simulink model "Vehicle_model_without_controller"  (R2024b)
settings: Solver=FixedStepAuto  StartTime=0  StopTime=1370  FixedStep=1  RelTol=1e-3
values from neighbouring files (symbols this model uses):
  Eff_2DLUT = [0.5417 0.5417 0.7 0.7908 0.8336 0.8638 0.9083 0.9278 0.9349 0.9437 0.9503 0.9475 ... (360 elements, 18x20)]    [MC_PM49.mat]    (also in motor_map_data.mat = [0.851419264642 0.851644655878 0.85189721745 0.852178660652 )
  Max_torque_1DLUT = [274.4 274.4 274.4 274.4 233.8 187 155.9 133.6 116.9 103.9 93.5 85 ... (18 elements, 18x1)]    [MC_PM49.mat]    (also in motor_map_data.mat = [300 300 300 300 300 300 300 300 300 300 300 290.819486922 .)
  motor_rpm = [0 500 1000 1500 2000 2500 3000 3500 4000 4500 5000 5500 ... (18 elements, 1x18)]    [MC_PM49.mat]    (also in motor_map_data.mat = [0 200 400 600 800 1000 1200 1400 1600 1800 2000 2200 ... (6)
  motor_trq = [-176.4 -156.8 -137.2 -117.6 -98 -78.4 -58.8 -39.2 -19.6 0 19.6 39.2 ... (20 elements, 20x1)]    [MC_PM49.mat]    (also in motor_map_data.mat = [-300 -288 -276 -264 -252 -240 -228 -216 -204 -192 -180 -168)
undefined symbols (not defined in the file or in its folder): DiscIntNeverNeededParam, eng_fuel_gps, eng_rpm_bp, eng_Tmax_tab, eng_tq_bp, LHV_kJ_g
settings Model: Creator=hesha  LastModifiedBy=yashp

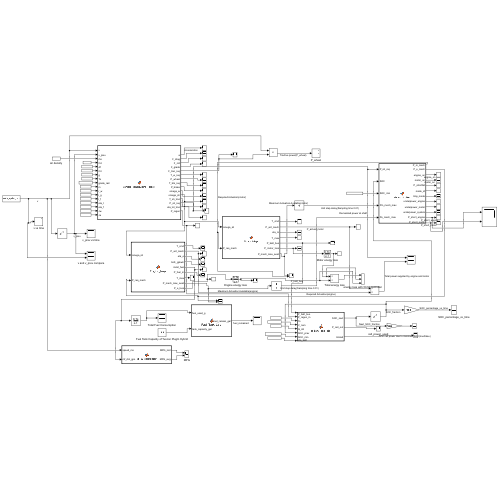
[thumbnail: Simulink's stored preview of the top-level diagram]
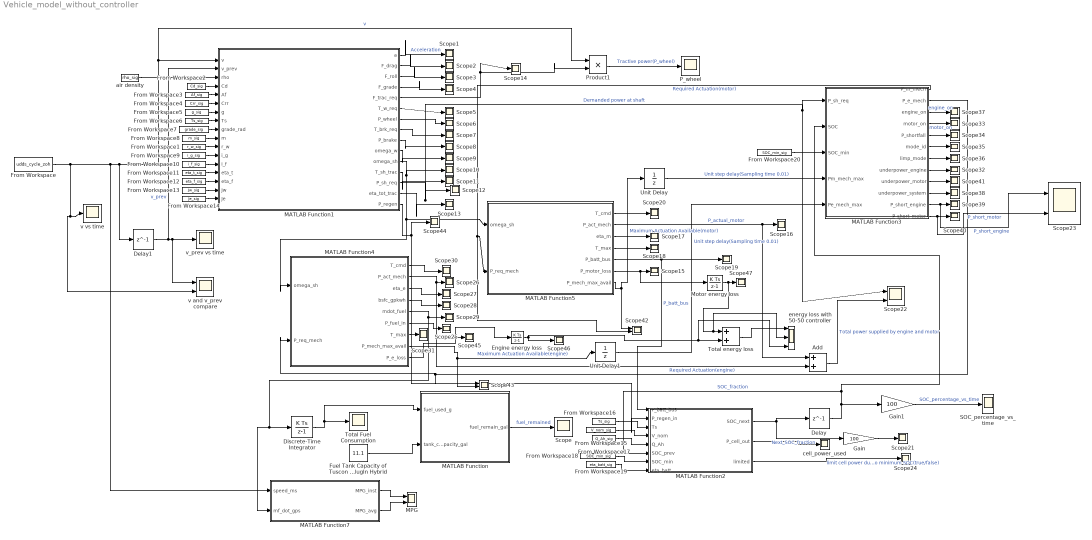
== system Vehicle_model_without_controller ==
  Add : Sum
  Delay : Delay  DelayLength=1  InitialCondition=0.8  InputProcessing=Columns as channels (frame based)
  Delay1 : Delay  DelayLength=1  InputProcessing=Columns as channels (frame based)
  Discrete-Time Integrator : DiscreteIntegrator  SampleTime=-1  ICPrevOutput=DiscIntNeverNeededParam  ICPrevScaledInput=DiscIntNeverNeededParam
  Engine energy loss : DiscreteIntegrator  SampleTime=-1  ICPrevOutput=DiscIntNeverNeededParam  ICPrevScaledInput=DiscIntNeverNeededParam
  From Workspace : FromWorkspace  VariableName=udds_cycle_zoh  OutDataTypeStr=double  SampleTime=-1  Interpolate=off  OutputAfterFinalValue=Setting to zero
  From Workspace1 : FromWorkspace  VariableName=r_w_sig  OutDataTypeStr=double  SampleTime=1  Interpolate=off  OutputAfterFinalValue=Setting to zero
  From Workspace10 : FromWorkspace  VariableName=i_f_sig  OutDataTypeStr=double  SampleTime=1  Interpolate=off  OutputAfterFinalValue=Setting to zero
  From Workspace11 : FromWorkspace  VariableName=eta_t_sig  OutDataTypeStr=double  SampleTime=1  Interpolate=off  OutputAfterFinalValue=Setting to zero
  From Workspace12 : FromWorkspace  VariableName=eta_f_sig  OutDataTypeStr=double  SampleTime=1  Interpolate=off  OutputAfterFinalValue=Setting to zero
  From Workspace13 : FromWorkspace  VariableName=Jw_sig  OutDataTypeStr=double  SampleTime=1  Interpolate=off  OutputAfterFinalValue=Setting to zero
  From Workspace14 : FromWorkspace  VariableName=Je_sig  OutDataTypeStr=double  SampleTime=1  Interpolate=off  OutputAfterFinalValue=Setting to zero
  From Workspace15 : FromWorkspace  VariableName=V_nom_sig  OutDataTypeStr=double  SampleTime=1  Interpolate=off  OutputAfterFinalValue=Setting to zero
  From Workspace16 : FromWorkspace  VariableName=Ts_sig  OutDataTypeStr=double  SampleTime=1  Interpolate=off  OutputAfterFinalValue=Setting to zero
  From Workspace17 : FromWorkspace  VariableName=Q_Ah_sig  OutDataTypeStr=double  SampleTime=1  Interpolate=off  OutputAfterFinalValue=Setting to zero
  From Workspace18 : FromWorkspace  VariableName=SOC_min_sig  OutDataTypeStr=double  SampleTime=1  Interpolate=off  OutputAfterFinalValue=Setting to zero
  From Workspace19 : FromWorkspace  VariableName=eta_batt_sig  OutDataTypeStr=double  SampleTime=1  Interpolate=off  OutputAfterFinalValue=Setting to zero
  From Workspace2 : FromWorkspace  VariableName=Cd_sig  OutDataTypeStr=double  SampleTime=1  Interpolate=off  OutputAfterFinalValue=Setting to zero
  From Workspace20 : FromWorkspace  VariableName=SOC_min_sig  OutDataTypeStr=double  SampleTime=1  Interpolate=off  OutputAfterFinalValue=Setting to zero
  From Workspace3 : FromWorkspace  VariableName=Af_sig  OutDataTypeStr=double  SampleTime=1  Interpolate=off  OutputAfterFinalValue=Setting to zero
  From Workspace4 : FromWorkspace  VariableName=Crr_sig  OutDataTypeStr=double  SampleTime=1  Interpolate=off  OutputAfterFinalValue=Setting to zero
  From Workspace5 : FromWorkspace  VariableName=g_sig  OutDataTypeStr=double  SampleTime=1  Interpolate=off  OutputAfterFinalValue=Setting to zero
  From Workspace6 : FromWorkspace  VariableName=Ts_sig  OutDataTypeStr=double  SampleTime=1  Interpolate=off  OutputAfterFinalValue=Setting to zero
  From Workspace7 : FromWorkspace  VariableName=grade_sig  OutDataTypeStr=double  SampleTime=1  Interpolate=off  OutputAfterFinalValue=Setting to zero
  From Workspace8 : FromWorkspace  VariableName=m_sig  OutDataTypeStr=double  SampleTime=1  Interpolate=off  OutputAfterFinalValue=Setting to zero
  From Workspace9 : FromWorkspace  VariableName=i_g_sig  OutDataTypeStr=double  SampleTime=1  Interpolate=off  OutputAfterFinalValue=Setting to zero
  Fuel Tank Capacity of Tuscon PlugIn Hybrid : Constant  Value=11.1
  Gain : Gain  Gain=100
  Gain1 : Gain  Gain=100
  MATLAB Function : MATLAB Function  TreatAsAtomicUnit=on
  MATLAB Function1 : MATLAB Function  TreatAsAtomicUnit=on
  MATLAB Function2 : MATLAB Function  TreatAsAtomicUnit=on
  MATLAB Function3 : MATLAB Function  TreatAsAtomicUnit=on
  MATLAB Function4 : MATLAB Function  TreatAsAtomicUnit=on
  MATLAB Function5 : MATLAB Function  TreatAsAtomicUnit=on
  MATLAB Function7 : MATLAB Function  TreatAsAtomicUnit=on
  MPG : Scope  NumInputPorts=2
  Motor energy loss : DiscreteIntegrator  SampleTime=-1  ICPrevOutput=DiscIntNeverNeededParam  ICPrevScaledInput=DiscIntNeverNeededParam
  P_wheel : Scope
  Product1 : Product
  SOC_percentage_vs_time : Scope
  Scope{,1..21,24..41,44..47} (44 alike) : Scope
  Scope{22..23,42..43} (4 alike) : Scope  NumInputPorts=2
  Total Fuel Consumption : Scope
  Total energy loss : Sum
  Unit Delay : UnitDelay  SampleTime=-1  HasFrameUpgradeWarning=on
  Unit Delay1 : UnitDelay  SampleTime=-1  HasFrameUpgradeWarning=on
  air density : FromWorkspace  VariableName=rho_sig  OutDataTypeStr=double  SampleTime=1  Interpolate=off  OutputAfterFinalValue=Setting to zero
  cell_power_used : Scope
  energy loss with 50-50 controller : Scope  NumInputPorts=3
  v and v_prev compare : Scope  NumInputPorts=2
  v vs time : Scope
  v_prev vs time : Scope
  wires:
  From Workspace/1 -> v and v_prev compare/2, v vs time/1, MATLAB Function7/1(speed_ms), Product1/1, MATLAB Function1/1(v), Delay1/1  "v"
  air density/1 -> MATLAB Function1/3(rho)
  From Workspace2/1 -> MATLAB Function1/4(Cd)
  From Workspace3/1 -> MATLAB Function1/5(Af)
  From Workspace4/1 -> MATLAB Function1/6(Crr)
  From Workspace5/1 -> MATLAB Function1/7(g)
  From Workspace6/1 -> MATLAB Function1/8(Ts)
  From Workspace8/1 -> MATLAB Function1/10(m)
  Delay1/1 -> MATLAB Function1/2(v_prev), v_prev vs time/1, v and v_prev compare/1  "v_prev"
  MATLAB Function1/5(F_trac_req) -> Scope14/1, Product1/2
  Product1/1 -> P_wheel/1  "Tractive power(P_wheel)"
  MATLAB Function1/1(a) -> Scope1/1  "Acceleration"
  From Workspace1/1 -> MATLAB Function1/11(r_w)
  From Workspace9/1 -> MATLAB Function1/12(i_g)
  From Workspace10/1 -> MATLAB Function1/13(i_f)
  From Workspace11/1 -> MATLAB Function1/14(eta_t)
  From Workspace12/1 -> MATLAB Function1/15(eta_f)
  From Workspace13/1 -> MATLAB Function1/16(Jw)
  From Workspace14/1 -> MATLAB Function1/17(Je)
  MATLAB Function1/2(F_drag) -> Scope2/1
  MATLAB Function1/3(F_roll) -> Scope3/1
  MATLAB Function1/4(F_grade) -> Scope4/1
  MATLAB Function1/6(T_w_req) -> Scope5/1
  MATLAB Function1/7(P_wheel) -> Scope6/1
  MATLAB Function1/8(T_brk_req) -> Scope7/1
  MATLAB Function1/9(P_brake) -> Scope8/1
  MATLAB Function1/10(omega_w) -> Scope9/1
  MATLAB Function1/11(omega_sh) -> Scope10/1, MATLAB Function4/1(omega_sh), MATLAB Function5/1(omega_sh)
  MATLAB Function1/12(T_sh_trac) -> Scope11/1
  MATLAB Function1/13(P_sh_req) -> MATLAB Function3/1(P_sh_req), Scope22/1, Scope12/1  "Demanded power at shaft"
  MATLAB Function1/14(eta_tot_trac) -> Scope13/1
  From Workspace16/1 -> MATLAB Function2/3(Ts)
  From Workspace7/1 -> MATLAB Function1/9(grade_rad)
  MATLAB Function3/1(P_m_mech) -> Scope42/2, MATLAB Function5/2(P_req_mech)  "Required Actuation(motor)"
  MATLAB Function3/2(P_e_mech) -> MATLAB Function4/2(P_req_mech), Scope43/1  "Required Actuation(engine)"
  MATLAB Function4/8(P_mech_max_avail) -> Scope43/2, Unit Delay1/1  "Maximum Actuation Available(engine)"
  MATLAB Function5/7(P_mech_max_avail) -> Unit Delay/1, Scope42/1  "Maximum Actuation Available(motor)"
  MATLAB Function2/1(SOC_next) -> Delay/1, Gain/1  "Next_SOC_fraction"
  Delay/1 -> Gain1/1, MATLAB Function3/2(SOC), MATLAB Function2/6(SOC_prev)  "SOC_fraction"
  MATLAB Function5/5(P_batt_bus) -> Scope19/1, MATLAB Function2/1(P_batt_bus)  "P_batt_bus"
  MATLAB Function5/2(P_act_mech) -> Add/1, Scope16/1  "P_actual_motor"
  MATLAB Function5/3(eta_m) -> Scope17/1
  MATLAB Function5/4(T_max) -> Scope18/1
  MATLAB Function5/1(T_cmd) -> Scope20/1
  Gain1/1 -> SOC_percentage_vs_time/1  "SOC_percentage_vs_time"
  MATLAB Function2/2(P_cell_out) -> cell_power_used/1
  MATLAB Function2/3(limited) -> Scope24/1  "limit cell power due to minimum SOC(true/false)"
  MATLAB Function4/3(eta_e) -> Scope27/1
  MATLAB Function4/2(P_act_mech) -> Add/2, Scope26/1
  MATLAB Function4/1(T_cmd) -> Scope30/1
  MATLAB Function4/4(bsfc_gpkwh) -> Scope28/1
  MATLAB Function4/5(mdot_fuel) -> Discrete-Time Integrator/1, MATLAB Function7/2(mf_dot_gps), Scope29/1
  MATLAB Function4/6(P_fuel_in) -> Scope25/1
  MATLAB Function4/7(T_max) -> Scope31/1
  From Workspace15/1 -> MATLAB Function2/4(V_nom)
  From Workspace17/1 -> MATLAB Function2/5(Q_Ah)
  From Workspace18/1 -> MATLAB Function2/7(SOC_min)
  From Workspace19/1 -> MATLAB Function2/8(eta_batt)
  From Workspace20/1 -> MATLAB Function3/3(SOC_min)
  Gain/1 -> Scope21/1
  Unit Delay1/1 -> MATLAB Function3/5(Pe_mech_max)  "Unit step delay(Sampling time 0.01)"
  Unit Delay/1 -> MATLAB Function3/4(Pm_mech_max)  "Unit step delay(Sampling time 0.01)"
  MATLAB Function3/3(engine_on) -> Scope37/1  "engine_on"
  MATLAB Function3/4(motor_on) -> Scope33/1  "motor_on"
  MATLAB Function3/5(P_shortfall) -> Scope34/1
  MATLAB Function3/6(mode_id) -> Scope35/1
  MATLAB Function3/7(limp_mode) -> Scope36/1
  MATLAB Function3/8(underpower_engine) -> Scope32/1
  MATLAB Function3/9(underpower_motor) -> Scope41/1
  MATLAB Function3/10(underpower_system) -> Scope38/1
  MATLAB Function3/11(P_short_engine) -> Scope23/1, Scope39/1  "P_short_engine"
  MATLAB Function3/12(P_short_motor) -> Scope23/2, Scope40/1  "P_short_motor"
  Discrete-Time Integrator/1 -> MATLAB Function/1(fuel_used_g), Total Fuel Consumption/1
  Add/1 -> Scope22/2  "Total power supplied by engine and motor"
  Fuel Tank Capacity of Tuscon PlugIn Hybrid/1 -> MATLAB Function/2(tank_capacity_gal)
  MATLAB Function/1(fuel_remain_gal) -> Scope/1  "fuel_remained"
  MATLAB Function4/9(P_e_loss) -> Scope45/1, Engine energy loss/1
  Engine energy loss/1 -> Scope46/1, Total energy loss/2, energy loss with 50-50 controller/3
  MATLAB Function5/6(P_motor_loss) -> Motor energy loss/1, Scope15/1
  Motor energy loss/1 -> energy loss with 50-50 controller/2, Total energy loss/1, Scope47/1
  Total energy loss/1 -> energy loss with 50-50 controller/1
  MATLAB Function7/1(MPG_inst) -> MPG/1
  MATLAB Function7/2(MPG_avg) -> MPG/2
  MATLAB Function1/15(P_regen) -> MATLAB Function2/2(P_regen_in), Scope44/1

== matlab function Vehicle_model_without_controller/MATLAB Function4 ==
  data: omega_sh input; T_cmd output; P_req_mech input; P_act_mech output; eta_e output; bsfc_gpkwh output; mdot_fuel output; P_fuel_in output; T_max output; P_mech_max_avail output; P_e_loss output; eng_rpm_bp parameter; eng_tq_bp parameter; eng_fuel_gps parameter; eng_Tmax_tab parameter; LHV_kJ_g parameter
function [T_cmd, P_act_mech, eta_e, bsfc_gpkwh, mdot_fuel, ...
          P_fuel_in, T_max, P_mech_max_avail, P_e_loss] = Engine_Map( ...
          omega_sh, P_req_mech, eng_rpm_bp, eng_tq_bp, eng_fuel_gps, eng_Tmax_tab, LHV_kJ_g)
%#codegen
% Engine_Map - FINAL REVISION
%   LUT-based engine model using ADVISOR FC_SI63_emis data.
%   FIX: Uses Fuel Rate Map (g/s) directly for P_fuel_in to avoid BSFC
%   instabilities near zero power.
%
% Inputs:
%   omega_sh    [rad/s]  shaft speed
%   P_req_mech  [W]      requested mechanical power (>=0)
%
% Outputs:
%   T_cmd              [Nm]   commanded engine torque
%   P_act_mech         [W]    actual mechanical power delivered
%   eta_e              [-]    engine efficiency
%   bsfc_gpkwh         [g/kWh] brake specific fuel consumption
%   mdot_fuel          [g/s]  fuel mass flow rate
%   P_fuel_in          [W]    fuel power input
%   T_max              [Nm]   max available torque at this speed
%   P_mech_max_avail   [W]    max mech power at this speed (T_max*omega)
%   P_e_loss           [W]    engine power loss (P_fuel_in - P_act_mech)
% -------------------------------------------------------------------------

%  1. Define constants and map parameters
rpm_bp      = eng_rpm_bp;     % [rpm]
tq_bp       = eng_tq_bp;      % [Nm]
fuel_tab    = eng_fuel_gps;   % [g/s]
Tmax_vec    = eng_Tmax_tab;   % [Nm]
LHV_kJ_g_c  = LHV_kJ_g;       % [kJ/g]

% --- Idle Constants (From FC_SI63_emis.m @ 701 RPM, 0 Nm) ---
idle_rpm               = 800;
idle_omega             = idle_rpm * 2*pi/60; % [rad/s]
idle_fuel_rate_fixed   = 0.1935;             % [g/s] (from fc_fuel_map[1,1])
idle_min_speed_in_map  = 701 * 2*pi/60;      % [rad/s]
% -------------------------------------------------------------------------

%  2. Requested power -> requested torque (with idle speed enforcement)
P_req_mech = max(P_req_mech, 0);          % Requested power must be >= 0

omega_safe = max(max(omega_sh, 1e-6), idle_omega);  % Enforce minimum running speed (idle)
rpm        = omega_safe * 60/(2*pi);

T_raw = P_req_mech / omega_safe; % [Nm] requested torque (Uses omega_safe for smooth behavior)

%  3. Max torque at this speed and Saturation
rpm_q_for_Tmax = clamp(rpm, rpm_bp(1), rpm_bp(end));
T_max = lin1D(rpm_bp, Tmax_vec, rpm_q_for_Tmax);   % [Nm]
T_max = max(T_max, 0);

% Saturate commanded torque: Must be >= 0 and <= T_max
T_cmd      = min(max(T_raw, 0), T_max);            % [Nm]
P_act_mech = T_cmd * omega_safe;                   % [W]

% Max mech power at this speed
P_mech_max_avail = T_max * omega_safe;             % [W]
% -------------------------------------------------------------------------

%  4. 2-D LUT for fuel rate (Using commanded T & current RPM)
tq_q   = clamp(T_cmd, tq_bp(1),  tq_bp(end));
rpm_q  = clamp(rpm,   rpm_bp(1), rpm_bp(end));

% Initial Lookups for fuel rate (mdot_fuel)
mdot_fuel_map   = bilinear2D(tq_bp, rpm_bp, fuel_tab, tq_q, rpm_q);   % [g/s]
% -------------------------------------------------------------------------

%  5. Efficiency and fuel power (Handling the Idle/Low-Power Region)
P_kW = P_act_mech / 1000;                    
idle_thr_kW = 1e-3;                          % ~1 W threshold

% Condition to trigger Idle Override: Very Low Power AND near the lowest operating speed
if (P_kW <= idle_thr_kW) && (omega_safe <= idle_min_speed_in_map * 1.05)
    
    % --- Idle Override ---
    mdot_fuel   = idle_fuel_rate_fixed;         % Fixed fuel consumption
    P_act_mech  = 0;                            % Actual mechanical power is zero at true idle
    eta_e       = 0;
    bsfc_gpkwh  = Inf;
    
    % P_fuel_in = mdot_fuel [g/s] * LHV_kJ_g [kJ/g] * 1000 [J/kJ] = [W]
    P_fuel_in   = mdot_fuel * LHV_kJ_g_c * 1000; % [W]
    
else
    % --- Normal Map Operation (using robust mdot_fuel lookup) ---
    mdot_fuel = mdot_fuel_map; % [g/s]

    % P_fuel_in = mdot_fuel [g/s] * LHV_kJ_g [kJ/g] * 1000 [J/kJ] = [W]
    P_fuel_in = mdot_fuel * LHV_kJ_g_c * 1000; % [W] 

    % Calculate efficiency (Power / Fuel Power)
    eta_e = P_act_mech / max(P_fuel_in, 1e-6); % Safe division

    % Calculate BSFC for logging/output (this will be the physically correct value)
    % BSFC = 3600 / (eta_e * LHV_kJ_g_c)
    bsfc_gpkwh = 3600 / max(eta_e * LHV_kJ_g_c, 1e-6);
    
    % Reset eta/bsfc if P_fuel_in is positive but P_act_mech is near zero
    if P_act_mech < 1 && mdot_fuel > 0
        eta_e = 0; 
        bsfc_gpkwh = Inf;
    end
end
% -------------------------------------------------------------------------

%  6. Power Loss Calculation (P_e_loss = P_fuel_in - P_act_mech)
P_e_loss = P_fuel_in - P_act_mech;  % [W] (Should now be in the 10^5 W range)

% Ensure positive loss (minor numerical safeguard)
P_e_loss = max(P_e_loss, 0);

end  % main function
% =========================================================================
% Helper functions (clamp, lin1D, bilinear2D remain unchanged)
% =========================================================================
function y = clamp(x,a,b)
% Clamp x into [a,b]
y = min(max(x,a),b);
end
function y = lin1D(xbp, ybp, xq)
% Simple 1-D linear interpolation (no fancy extrapolation)
n = numel(xbp);
if xq <= xbp(1)
    y = ybp(1);
elseif xq >= xbp(end)
    y = ybp(end);
else
    i = 1;
    for k = 2:n
        if xq < xbp(k)
            i = k - 1;
            break;
        end
    end
    t = (xq - xbp(i)) / (xbp(i+1) - xbp(i));
    y = (1 - t)*ybp(i) + t*ybp(i+1);
end
end
function z = bilinear2D(xbp, ybp, tab, xq, yq)
% Bilinear interpolation on regular grid
% xbp: torque axis (1D)  -> columns of tab
% ybp: rpm axis   (1D)   -> rows of tab
Nx = numel(xbp);
Ny = numel(ybp);
% --- x index (torque) ---
if xq <= xbp(1)
    i = 1; tx = 0;
elseif xq >= xbp(end)
    i = Nx - 1; tx = 1;
else
    i = 1;
    for k = 2:Nx
        if xq < xbp(k)
            i = k - 1;
            break;
        end
    end
    tx = (xq - xbp(i)) / (xbp(i+1) - xbp(i));
end
% --- y index (rpm) ---
if yq <= ybp(1)
    j = 1; ty = 0;
elseif yq >= ybp(end)
    j = Ny - 1; ty = 1;
else
    j = 1;
    for k = 2:Ny
        if yq < ybp(k)
            j = k - 1;
            break;
        end
    end
    ty = (yq - ybp(j)) / (ybp(j+1) - ybp(j));
end
% Corner values
f11 = tab(j   , i   );
f12 = tab(j+1 , i   );
f21 = tab(j   , i+1 );
f22 = tab(j+1 , i+1 );
% Basic NaN clean-up in masked region
if isnan(f11), f11 = f12; end
if isnan(f22), f22 = f21; end
if isnan(f21), f21 = f22; end
if isnan(f12), f12 = f11; end
% Bilinear interpolation
z = (1-tx)*(1-ty)*f11 + tx*(1-ty)*f21 + ...
    (1-tx)*ty*f12     + tx*ty*f22;
end

== matlab function Vehicle_model_without_controller/MATLAB Function5 ==
  data: omega_sh input; T_cmd output; P_req_mech input; P_act_mech output; eta_m output; T_max output; P_batt_bus output; P_motor_loss output; P_mech_max_avail output; motor_rpm parameter; motor_trq parameter; Eff_2DLUT parameter; Max_torque_1DLUT parameter
function [T_cmd, P_act_mech, eta_m, T_max, ...
          P_batt_bus, P_motor_loss, P_mech_max_avail] = Motor_Map( ...
          omega_sh, P_req_mech, motor_rpm, motor_trq, Eff_2DLUT, Max_torque_1DLUT)
%#codegen
% Motor_Map
%   LUT-based motor model using ADVISOR MC_PM49 data.
%   Traction only (P_req_mech >= 0).
%
% Inputs:
%   omega_sh    [rad/s] shaft speed
%   P_req_mech  [W]     requested mechanical power
%
% Outputs:
%   T_cmd              [Nm] commanded motor torque
%   P_act_mech         [W]  actual mechanical power delivered
%   eta_m              [-]  motor efficiency
%   T_max              [Nm] max motoring torque at this speed
%   P_batt_bus         [W]  DC bus power drawn from battery
%   P_motor_loss       [W]  motor+inverter loss
%   P_mech_max_avail   [W]  max mech power at this speed (T_max*omega)

% -------------------------------------------------------------------------
% 1. Treat LUTs from workspace as constants
% -------------------------------------------------------------------------
rpm_bp   = motor_rpm(:);          % [rpm], Nr x 1
tq_bp    = motor_trq(:);          % [Nm],  Nt x 1
eff_tab  = Eff_2DLUT;             % [--],  Nr x Nt
Tmax_vec = Max_torque_1DLUT(:);   % [Nm],  Nr x 1

% -------------------------------------------------------------------------
% 2. Guards and basic conversions
% -------------------------------------------------------------------------
% Traction only
if P_req_mech < 0
    P_req_mech = 0;
end

omega_safe = max(omega_sh, 1e-6);             % [rad/s], avoid /0
rpm        = omega_safe * 60/(2*pi);          % [rpm]

% -------------------------------------------------------------------------
% 3. Requested torque and max torque
% -------------------------------------------------------------------------
T_raw = P_req_mech / omega_safe;              % [Nm] requested torque

% Max torque vs speed (1-D LUT)
rpm_q_for_Tmax = clamp(rpm, rpm_bp(1), rpm_bp(end));
T_max = lin1D(rpm_bp, Tmax_vec, rpm_q_for_Tmax);  % [Nm]
T_max = max(T_max, 0);

% Saturate torque command
T_cmd      = min(max(T_raw, 0), T_max);       % [Nm]
P_act_mech = T_cmd * omega_safe;              % [W]

% Max mech power available
P_mech_max_avail = T_max * omega_safe;        % [W]

% -------------------------------------------------------------------------
% 4. Efficiency lookup (2-D LUT)
% -------------------------------------------------------------------------
tq_q  = clamp(T_cmd, tq_bp(1), tq_bp(end));
rpm_q = clamp(rpm,   rpm_bp(1), rpm_bp(end));

eta_m = bilinear2D(tq_bp, rpm_bp, eff_tab, tq_q, rpm_q);  % 0..1
eta_m = min(max(eta_m, 1e-3), 0.999);        % numeric guard

% -------------------------------------------------------------------------
% 5. Electrical power and losses
% -------------------------------------------------------------------------
if P_act_mech <= 1e-6
    P_batt_bus   = 0;
    P_motor_loss = 0;
else
    P_batt_bus   = P_act_mech / eta_m;       % [W]
    P_motor_loss = P_batt_bus - P_act_mech;  % [W]
end

end % main function

% =========================================================================
% Helper functions
% =========================================================================

function y = clamp(x,a,b)
y = min(max(x,a),b);
end

function y = lin1D(xbp, ybp, xq)
% 1-D linear interpolation with simple end extrapolation
n = numel(xbp);

if xq <= xbp(1)
    y = ybp(1) + (ybp(2)-ybp(1))*(xq-xbp(1))/(xbp(2)-xbp(1));
elseif xq >= xbp(end)
    y = ybp(end-1) + (ybp(end)-ybp(end-1))*(xq-xbp(end-1))/(xbp(end)-xbp(end-1));
else
    i = 1;
    for k = 2:n
        if xq < xbp(k)
            i = k-1;
            break;
        end
    end
    t = (xq - xbp(i))/(xbp(i+1)-xbp(i));
    y = (1-t)*ybp(i) + t*ybp(i+1);
end
end

function z = bilinear2D(xbp, ybp, tab, xq, yq)
% Bilinear interpolation on regular grid
% xbp: torque axis (columns), ybp: speed axis (rows)
Nx = numel(xbp);
Ny = numel(ybp);

% --- x (torque) index ---
if xq <= xbp(1)
    i = 1; tx = 0;
elseif xq >= xbp(end)
    i = Nx-1; tx = 1;
else
    i = 1;
    for k = 2:Nx
        if xq < xbp(k)
            i = k-1;
            break;
        end
    end
    tx = (xq - xbp(i))/(xbp(i+1)-xbp(i));
end

% --- y (speed) index ---
if yq <= ybp(1)
    j = 1; ty = 0;
elseif yq >= ybp(end)
    j = Ny-1; ty = 1;
else
    j = 1;
    for k = 2:Ny
        if yq < ybp(k)
            j = k-1;
            break;
        end
    end
    ty = (yq - ybp(j))/(ybp(j+1)-ybp(j));
end

% Corner values
f11 = tab(j   , i   );
f12 = tab(j+1 , i   );
f21 = tab(j   , i+1 );
f22 = tab(j+1 , i+1 );

% Simple NaN handling
if isnan(f11), f11 = f12; end
if isnan(f22), f22 = f21; end
if isnan(f21), f21 = f22; end
if isnan(f12), f12 = f11; end

% Bilinear blend
z = (1-tx)*(1-ty)*f11 + tx*(1-ty)*f21 + ...
    (1-tx)*ty*f12     + tx*ty*f22;
end

== matlab function Vehicle_model_without_controller/MATLAB Function7 ==
  data: speed_ms input; MPG_inst output; mf_dot_gps input; MPG_avg output
function [MPG_inst, MPG_avg] = MPG_calculator(speed_ms, mf_dot_gps)

MS_TO_MPH = 2.236936;
G_PER_GAL = 2819;

speed_mph = speed_ms * MS_TO_MPH;
fuel_gal_per_hr = (mf_dot_gps * 3600) / G_PER_GAL;

if fuel_gal_per_hr == 0
    MPG_inst = 0;
else
    MPG_inst = speed_mph / fuel_gal_per_hr;
end

persistent MPG_sum count
if isempty(MPG_sum)
    MPG_sum = 0;
    count = 0;
end

MPG_sum = MPG_sum + MPG_inst;
count = count + 1;

MPG_avg = MPG_sum / count;

end

== matlab function Vehicle_model_without_controller/MATLAB Function1 ==
  data: a output; F_drag output; F_roll output; F_grade output; v input; F_trac_req output; v_prev input; rho input; Cd input; Af input; Crr input; g input; Ts input; grade_rad input; m input; r_w input; i_g input; i_f input; eta_t input; eta_f input; Jw input; Je input; T_w_req output; P_wheel output; T_brk_req output; P_brake output; omega_w output; omega_sh output; T_sh_trac output; P_sh_req output; eta_tot_trac output; P_regen output
function [a, F_drag, F_roll, F_grade, F_trac_req, T_w_req, P_wheel, T_brk_req, P_brake, omega_w, omega_sh, T_sh_trac, P_sh_req, eta_tot_trac, P_regen] = vehicle_longitudinal_block(v, v_prev, rho, Cd, Af, Crr, g, Ts, grade_rad, m, r_w, i_g, i_f, eta_t, eta_f, Jw, Je)
% Vehicle longitudinal dynamics (no regen) with separate gearbox & final-drive
% efficiencies. Positive power = traction; braking is hydraulic only.
%
% P_wheel = eta_tot_trac * P_shaft,  where eta_tot_trac = eta_t * eta_f
% i_tot   = i_g * i_f

% --- guards ---
Ts  = max(Ts, 1e-9);
r_w = max(r_w, 1e-6);
i_tot = max(i_g*i_f, 1e-6);
eta_t = min(max(eta_t ,1e-3), 1.0);
eta_f = min(max(eta_f ,1e-3), 1.0);
eta_tot_trac = eta_t * eta_f;

% --- kinematics ---
a           = (v - v_prev)/Ts;
omega_w     = v / r_w; % angular speed
omega_w_dot = a / r_w; % aplha or angular acceleration wheel

% --- resistive forces ---
F_drag  = 0.5 * rho * Cd * Af * v * abs(v);
F_roll  = Crr * m * g * cos(grade_rad);
F_grade = m   * g * sin(grade_rad);

% --- inertial terms ---
F_inert_mass = m * a;
T_inert_mass = F_inert_mass * r_w;
T_inert_rot  = Jw*omega_w_dot + (i_tot^2)*Je*omega_w_dot;

% --- wheel torque/force & powers ---
T_res_w    = (F_drag + F_roll + F_grade)*r_w;
T_w_req    = T_inert_mass + T_inert_rot + T_res_w;
F_trac_req = T_w_req / r_w;
P_wheel    = F_trac_req * v;

% braking (no regen)
T_brk_req = max(-T_w_req, 0);
P_brake   = max(-P_wheel, 0);

% --- map to shaft for traction only ---
omega_sh = i_tot * omega_w; % angular speed of clutch
% Initialize the new output P_regen
P_regen = 0.0;

if P_wheel > 0
    % P_shaft before devices (engine/motor input)
    P_sh_req  = P_wheel / eta_tot_trac; % Power required at clutch
    wsh_safe  = max(omega_sh, 1e-6);
    T_sh_trac = P_sh_req / wsh_safe;           % info/logging % Torque required at clutch
else
    P_sh_req  = 0; % Power required at clutch
    T_sh_trac = 0; % Torque required at clutch
    % New: P_regen output holds the negative wheel power available for recapture
    if P_wheel < 0 
        P_regen = P_wheel; % P_regen is negative (power flowing OUT of vehicle to battery)
    end
end

== matlab function Vehicle_model_without_controller/MATLAB Function ==
  data: fuel_used_g input; fuel_remain_gal output; tank_capacity_gal input
function fuel_remain_gal = Fuel_Tank_Calc(fuel_used_g, tank_capacity_gal)
%#codegen
% Calculates remaining fuel in tank (in gallons)
%
% Inputs:
%   fuel_used_g        - Total fuel used [g]
%   tank_capacity_gal  - Tank capacity [US gallons]
%
% Output:
%   fuel_remain_gal    - Remaining fuel [US gallons]
%
% Assumptions:
%   Gasoline density = 0.745 kg/L

    % --- constants ---
    rho_gasoline = 0.745;       % [kg/L]
    L_per_gal    = 3.78541;     % [L/gal]

    % --- convert used fuel ---
    fuel_used_kg = fuel_used_g / 1000;          % g → kg
    fuel_used_L  = fuel_used_kg / rho_gasoline; % kg → L
    fuel_used_gal = fuel_used_L / L_per_gal;    % L → gal

    % --- remaining fuel ---
    fuel_remain_gal = max(tank_capacity_gal - fuel_used_gal, 0); % ensure non-negative

end

== matlab function Vehicle_model_without_controller/MATLAB Function2 ==
  data: P_batt_bus input; P_regen_in input; SOC_next output; Ts input; V_nom input; Q_Ah input; SOC_prev input; SOC_min input; eta_batt input; P_cell_out output; limited output
function [SOC_next, P_cell_out, limited] = battery_soc_eta(P_batt_bus, P_regen_in, Ts, V_nom, Q_Ah, SOC_prev, SOC_min, eta_batt)
% Power-based SOC integrator with battery efficiency.
% P_batt_bus >= 0 is DC bus draw (Traction).
% P_regen_in <= 0 is DC bus input (Regen).

% --- Guards and Constants ---
Ts       = max(Ts, 1e-9);
E_nom    = max(V_nom*Q_Ah*3600, 1.0);   % [J]
eta_batt = min(max(eta_batt, 1e-3), 1.0); % Discharge efficiency

% --- Updated: Regen Efficiency ---
eta_regen = 0.65;
SOC_max   = 0.80; % Assuming a safe max limit for clipping

% --- Determine Net Power Flow & Apply Correct Efficiency ---
% We rely on the fact that either P_batt_bus or P_regen_in will be near zero
% based on the vehicle dynamics block output.

if P_regen_in < 0
    % CASE 1: CHARGING (Regeneration)
    % P_regen_in is negative power generated by motor.
    P_bus_net = P_regen_in;
    % Chemical power entering cells is less negative than bus power (P_cell is negative)
    P_cell = P_bus_net * eta_regen;
else
    % CASE 2: DISCHARGING (Traction or Coast)
    % P_bus must be P_batt_bus (which is positive or zero)
    P_bus = max(P_batt_bus, 0);             % ensures no charging if P_regen_in was zero/positive
    P_cell = P_bus / eta_batt;               % chemical power leaving cells (Positive)
end

% -------------------------------------------------------------------------
% Integrate and Apply Limits
% -------------------------------------------------------------------------
% proposed update: dSOC is now signed based on P_cell
dSOC = (P_cell * Ts) / E_nom;
SOC_tmp = SOC_prev - dSOC; % P_cell > 0 decreases SOC; P_cell < 0 increases SOC

limited = false;

if P_cell > 0 && SOC_tmp < SOC_min 
    % --- LIMIT 1: DISCHARGE CLIPPING (P_cell is positive) ---
    % scale draw to just reach SOC_min this step
    allowed_E = (SOC_prev - SOC_min) * E_nom;       % [J]
    P_cell_allowed = allowed_E / Ts;                % [W] (Positive)
    scale = P_cell_allowed / max(P_cell,1e-9);
    
    P_cell_out = P_cell * min(scale,1.0);
    SOC_next   = SOC_prev - (P_cell_out*Ts)/E_nom;
    limited    = true;

elseif P_cell < 0 && SOC_tmp > SOC_max
    % --- LIMIT 2: CHARGE CLIPPING (P_cell is negative) ---
    % scale charge to just reach SOC_max this step
    allowed_E_charge = (SOC_max - SOC_prev) * E_nom;  % [J]
    P_cell_allowed_neg = -allowed_E_charge / Ts;      % [W] (Negative)
    
    % Scale factor calculation (both P_cell and P_cell_allowed_neg are negative)
    scale = P_cell_allowed_neg / min(P_cell, -1e-9); 
    
    P_cell_out = P_cell * min(scale, 1.0); % P_cell_out remains negative
    SOC_next   = SOC_prev - (P_cell_out*Ts)/E_nom;
    limited    = true;

else
    % --- NO CLIPPING ---
    P_cell_out = P_cell;
    SOC_next   = SOC_tmp;
end
end

== matlab function Vehicle_model_without_controller/MATLAB Function3 ==
  data: P_sh_req input; P_m_mech output; SOC input; SOC_min input; Pm_mech_max input; Pe_mech_max input; P_e_mech output; engine_on output; motor_on output; P_shortfall output; mode_id output; limp_mode output; underpower_engine output; underpower_motor output; underpower_system output; P_short_engine output; P_short_motor output
function [P_m_mech, P_e_mech, engine_on, motor_on, ...
          P_shortfall, mode_id, limp_mode, ...
          underpower_engine, underpower_motor, underpower_system, ...
          P_short_engine, P_short_motor] = ...
    rb_controller(P_sh_req, SOC, SOC_min, Pm_mech_max, Pe_mech_max)
% Minimal rule-based controller (no regen/charging)
% ---------------------------------------------------------------
% Power split (all powers are MECHANICAL at transmission input):
%   - If P_req <= 0: both off (braking hydraulic)
%   - If SOC <= SOC_min: ENGINE ONLY, capped by Pe_mech_max
%   - Else: 50/50 split, each capped; NO redistribution
%
% Additional monitoring outputs:
%   limp_mode         : engine-only AND unmet demand
%   underpower_engine : engine hit its cap for the requested share/role
%   underpower_motor  : motor  hit its cap for the requested share/role
%   underpower_system : total unmet demand (P_shortfall > 0)
%   P_short_engine    : unmet portion attributable to engine cap
%   P_short_motor     : unmet portion attributable to motor cap
%
% Notes:
% - In engine-only mode, P_short_engine = max(P_req - Pe_mech_max, 0), motor = 0.
% - In 50/50 mode, P_short_engine = max(0.5*P_req - Pe_mech_max, 0),
%   and P_short_motor = max(0.5*P_req - Pm_mech_max, 0).
%   Since there's no redistribution, P_shortfall = P_short_engine + P_short_motor.

% ---- guards ----
P_req       = max(P_sh_req, 0);
Pm_mech_max = max(Pm_mech_max, 0);
Pe_mech_max = max(Pe_mech_max, 0);

% defaults
P_m_mech = 0; 
P_e_mech = 0; 
engine_on = false; 
motor_on  = false;
mode_id   = 0;

P_shortfall    = 0;
limp_mode      = false;
underpower_engine = false;
underpower_motor  = false;
underpower_system = false;
P_short_engine = 0;
P_short_motor  = 0;

% ---- case 1: braking or idle ----
if P_req <= 1e-9
    return;
end

% ---- case 2: SOC protection (engine only) ----
if SOC <= SOC_min
    % engine contribution
    P_e_mech      = min(P_req, Pe_mech_max);
    P_m_mech      = 0;

    % shortfalls (motor is off by rule)
    P_short_engine   = max(P_req - Pe_mech_max, 0);
    P_short_motor    = 0;
    P_shortfall      = P_short_engine;  % all shortfall stems from engine cap here

    % flags
    underpower_engine = P_short_engine > 1e-6;
    underpower_motor  = false;
    underpower_system = P_shortfall > 1e-6;
    limp_mode         = underpower_system;  % engine-only & unmet demand

    engine_on  = P_e_mech > 1e-6;
    motor_on   = false;
    mode_id    = limp_mode * 4 + (~limp_mode) * 3; % 3=engine-only, 4=limited
    return;
end

% ---- case 3: EV-allowed region (50/50 split, no redistribution) ----
share_e_req = 0.5 * P_req;
share_m_req = 0.5 * P_req;

% apply per-side caps
P_e_mech = min(share_e_req, Pe_mech_max);
P_m_mech = min(share_m_req, Pm_mech_max);

% component shortfalls due to their own caps
P_short_engine = max(share_e_req - Pe_mech_max, 0);
P_short_motor  = max(share_m_req - Pm_mech_max, 0);

% total unmet demand (no redistribution)
P_shortfall    = P_short_engine + P_short_motor;

% flags
underpower_engine = P_short_engine > 1e-6;
underpower_motor  = P_short_motor  > 1e-6;
underpower_system = P_shortfall    > 1e-6;
limp_mode         = false; % by definition only in engine-only SOC protection

engine_on = P_e_mech > 1e-6;
motor_on  = P_m_mech > 1e-6;

if engine_on && motor_on
    mode_id = underpower_system * 4 + (~underpower_system) * 2; % 2=hybrid, 4=limited
elseif engine_on
    mode_id = underpower_system * 4 + (~underpower_system) * 3; % 3=engine-only
elseif motor_on
    mode_id = underpower_system * 4 + (~underpower_system) * 1; % 1=EV
else
    mode_id = 0;
end
